simulink model "Coil_Gun_Simulations"  (R2020b)
settings: Solver=VariableStepAuto  StartTime=0.0  StopTime=1
model workspace (MAT data in the model file):
  Coil_Diameter = Simulink.Parameter
  Coil_Diameter.Value = 10
  Coil_Diameter.DataType = 'auto'
  Coil_Diameter.DocUnits = 'mm'
  Coil_Diameter.Dimensions = [1 1]
  Coil_Length = Simulink.Parameter
  Coil_Length.Value = 5
  Coil_Length.DataType = 'auto'
  Coil_Length.DocUnits = 'mm'
  Coil_Length.Dimensions = [1 1]
  Coil_Turns = Simulink.Parameter
  Coil_Turns.Value = 20
  Coil_Turns.DataType = 'auto'
  Coil_Turns.Dimensions = [1 1]
  Projectile_Density = Simulink.Parameter
  Projectile_Density.Value = 7850
  Projectile_Density.DataType = 'auto'
  Projectile_Density.DocUnits = 'kg/m^3'
  Projectile_Density.Dimensions = [1 1]
  Projectile_Diameter = Simulink.Parameter
  Projectile_Diameter.Value = 5
  Projectile_Diameter.DataType = 'auto'
  Projectile_Diameter.DocUnits = 'mm'
  Projectile_Diameter.Dimensions = [1 1]
  Projectile_Length = Simulink.Parameter
  Projectile_Length.Value = 5
  Projectile_Length.DataType = 'auto'
  Projectile_Length.DocUnits = 'mm'
  Projectile_Length.Dimensions = [1 1]
  u0 = Simulink.Parameter
  u0.Value = 1.256636e-06
  u0.DataType = 'auto'
  u0.DocUnits = 'N/A^2'
  u0.Dimensions = [1 1]
libraries: fl_lib x5, nesl_utility x4, ee_lib x3
settings Model: OrderedModelArguments=off  Creator=hanso  LastModifiedBy=hanso
settings SolverCC: ZeroCrossAlgorithm=Adaptive

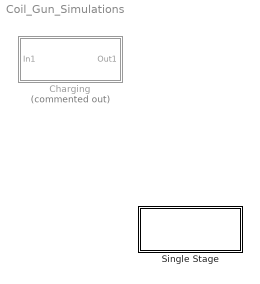
== system Coil_Gun_Simulations ==
  Charging : Subsystem  Commented=on
  Single Stage : Subsystem

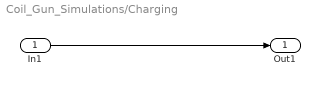
== system Coil_Gun_Simulations/Charging ==
  In1 : Inport
  Out1 : Outport
  wires:
  In1/1 -> Out1/1

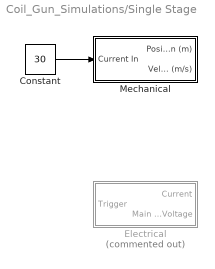
== system Coil_Gun_Simulations/Single Stage ==
  Constant : Constant  Value=30
  Electrical : Subsystem  Commented=on
  Mechanical : Subsystem
  wires:
  Constant/1 -> Mechanical/1(Current In)

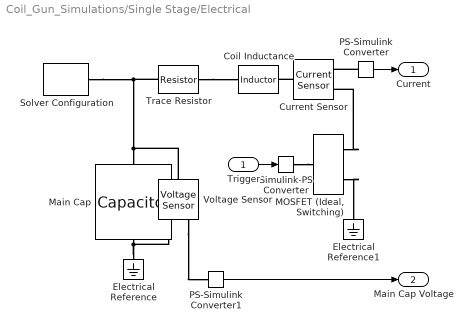
== system Coil_Gun_Simulations/Single Stage/Electrical ==
  Trigger : Inport
  Coil Inductance : ee_lib/Passive/Inductor  l=1e-03 H  L_tol=10  enable_L_tol=0  tol_distribution=1  nSigma=4  r=0 Ohm  g=1e-9 1/Ohm  enable_operating_limits=0  operating_limit_action=2  max_working_current=1 A  power_rating=1 W  enable_faults=0  fault_action=1  lambdaPercent=50  k_faulted=0.9999  turnsShort=0  openCct=0  groundShort=0  groundShortG=0 1/Ohm  tau_fault=1e-3 s  enable_temporal_fault=0  t_fault=1 s  enable_behavioral_fault=0  max_permissible_voltage=100 V  n_fail_on_voltage=1  max_permissible_current=1 A  t_fail_on_current=1 s  i_L_specify=off  i_L_priority=High  i_L=0 A  i_L_nominal_specify=off  i_L_nominal_unit=A  i_L_nominal_value=1
  Current Sensor : fl_lib/Electrical/Electrical Sensors/Current Sensor
  Electrical Reference : fl_lib/Electrical/Electrical Elements/Electrical Reference
  Electrical Reference1 : fl_lib/Electrical/Electrical Elements/Electrical Reference
  "MOSFET (Ideal, Switching)" : ee_lib/Semiconductors & Converters/MOSFET (Ideal, Switching)  Rds=0.01 Ohm  Goff=1e-6 1/Ohm  Vth=2 V  diode_param=ee.enum.converters.protectiondiode.none  diode_Vf=0.8 V  diode_Ron=0.001 Ohm  diode_Goff=1e-5 1/Ohm  diode_C=50e-9 F  diode_iRM=-235 A  diode_iF=300 A  diode_idot=-50 A/us  diode_trr_param=ee.enum.converters.diodetrr.trr_factor  diode_trr_factor=3  diode_trr=15 us  diode_Qrr=1500 s*uA  thermal_loss_option=ee.enum.converters.thermalLossOption.constantvalues  Von_data=[0, 1.1, 1.3, 1.45, 1.75, 2.25, 2.7; 0, 1, 1.15, 1.35, 1.7, 2.35, 3] V  Eon_data=[0, .29, 1.43, 2.86, 5.71, 13.14, 22.86; 0, .57, 2.63, 5.14, 10.29, 20.57, 30.29] * 1e-3 J  Eoff_data=[0, .21, 1.07, 2.14, 4.29, 9.86, 17.14; 0, .43, 1.97, 3.86, 7.71, 15.43, 22.71] * 1e-3 J  Tj=[298.15, 398.15] K  Iout_data=[0, 10, 50, 100, 200, 400, 600] A  Eon_scalar=22.86e-3 J  Eoff_scalar=17.14e-3 J  Voff=300 V  Iout_scalar=600 A  diodeModelType=ee.enum.converters.diodeModelType.pwl  diode_IfMat=[.07, .12, .19, 1.75, 4.24, 7.32, 11.2; .16, .3, .72, 2.14, 4.02, 6.35, 9.12] A  diode_TjVec=[25, 125] degC  diode_VfVec=[.5, .7, .9, 1.3, 1.7, 2.1, 2.5] V  thermal_network_parameterization=ee.enum.thermalNetworkTopology.external  Rth=[.03, .2] K/W  Rth_Foster=[.03, .2] K/W  thermal_mass_parameterization=ee.enum.thermalNetwork.timeconstant  thermal_mass=[3, 25] J/K  thermal_mass_Foster=[33, 50] J/K  thermal_time_constant=[.1, 5] s  thermal_time_constant_Foster=[1, 10] s  thermal_mass_initial_temperatures=[25, 25] degC  junction_thermal_mass=0.1 J/K  Tau=1e-4 s  vT_specify=off  vT_priority=None  vT=0 V  vT_nominal_specify=off  vT_nominal_unit=V  vT_nominal_value=1  Qj_specify=off  Qj_priority=None  Qj=0 W  Qj_nominal_specify=off  Qj_nominal_unit=W  Qj_nominal_value=1  junction_temperature_specify=off  junction_temperature_priority=None  junction_temperature=25 degC  junction_temperature_nominal_specify=off  junction_temperature_nominal_unit=degC  junction_temperature_nominal_value=1
  Main Cap : ee_lib/Passive/Capacitor  cap_option=0  c=2400e-6 F  Cvec=[1e-05, 1e-06] F  Vvec=[0, 10] V  CV_table_symmetry=1  f_vec=[1, 10] kHz  DFext_vec=[.8, 1.2]  C_tol=5  enable_C_tol=0  tol_distribution=1  nSigma=4  r=1e-6 Ohm  g=0 1/Ohm  averaging_period=0 s  enable_operating_limits=0  operating_limit_action=2  max_working_voltage_range=[-25, 25] V  power_rating=1 W  enable_faults=0  fault_action=1  Cscale_faulted=100  R_faulted=1e-3 Ohm  G_faulted=0 1/Ohm  tau_fault=1e-3 s  enable_temporal_fault=0  t_fault=1 s  enable_behavioral_fault=0  max_permissible_voltage_range=[-100, 100] V  t_fail_on_voltage=1 s  i_specify=off  i_priority=None  i=0 A  i_nominal_specify=off  i_nominal_unit=A  i_nominal_value=1  v_specify=off  v_priority=None  v=10 V  v_nominal_specify=off  v_nominal_unit=V  v_nominal_value=1  vc_specify=on  vc_priority=High  vc=10 V  vc_nominal_specify=off  vc_nominal_unit=V  vc_nominal_value=1
  PS-Simulink Converter : nesl_utility/PS-Simulink Converter  PhysicalDomain=network_engine_domain  SubClassName=ps_output  LeftPortType=input  RightPortType=output  PseudoPeriodic=off  Frequencies=[]  Unit=inherit  AffineConversion=off
  PS-Simulink Converter1 : nesl_utility/PS-Simulink Converter  PhysicalDomain=network_engine_domain  SubClassName=ps_output  LeftPortType=input  RightPortType=output  PseudoPeriodic=off  Frequencies=[]  Unit=inherit  AffineConversion=off
  Simulink-PS Converter : nesl_utility/Simulink-PS Converter  PhysicalDomain=network_engine_domain  SubClassName=ps_input  LeftPortType=input  RightPortType=output  PseudoPeriodic=off  Frequencies=[]  NoiseDistribution=none  NoiseParameters=[]  Unit=1  AffineConversion=off  FilteringAndDerivatives=provide  SimscapeFilterOrder=1  InputFilterTimeConstant=0.001  UdotUserProvided=0
  Solver Configuration : nesl_utility/Solver Configuration  PhysicalDomain=network_engine_domain  SubClassName=solver  LeftPortType=input  RightPortType=generic  Tones=[]  Harmonics=[]  SimulateNoise=off  Profile=off  UseLocalSampling=off  EnableSwitchedLinearOptims=on  FrequencyDomain=off  UseCCode=off  RelTol=0.001  AbsTol=1e-06  MinStep=1e-09  ToWorkspace=off  RevertToSquareIcSolve=off  NumHomotopyIterations=100  PhasorMode=off  PhasorModeNumHarmonics=1  DoDC=off  ResidualTolerance=1e-09  UseLocalSolver=off  LocalSolverChoice=NE_TRAPEZOIDAL_ADVANCER  LocalSolverSampleTime=1e-6  DoFixedCost=off  MaxNonlinIter=3  MaxModeIter=2  ComputeImpulses=off  ImpulseIterations=2  LinearAlgebra=auto  EquationFormulation=NE_TIME_EF  DelaysMemoryBudget=1024  AutomaticFiltering=off  FilteringTimeConstant=0.001  PartitionStorageMethod=AS_NEEDED  PartitionMemoryBudget=1024  PartitionMethod=ROBUST
  Trace Resistor : fl_lib/Electrical/Electrical Elements/Resistor  R=1 Ohm  i_specify=off  i_priority=None  i=0 A  i_nominal_specify=off  i_nominal_unit=A  i_nominal_value=1  v_specify=off  v_priority=None  v=0 V  v_nominal_specify=off  v_nominal_unit=V  v_nominal_value=1
  Voltage Sensor : fl_lib/Electrical/Electrical Sensors/Voltage Sensor
  Current : Outport
  Main Cap Voltage : Outport  Port=2
  wires:
  PS-Simulink Converter/1 -> Current/1
  PS-Simulink Converter1/1 -> Main Cap Voltage/1
  Trigger/1 -> Simulink-PS Converter/1
  connections:
  Solver Configuration/RConn1 -- Trace Resistor/LConn1 -- Voltage Sensor/LConn1 -- Main Cap/LConn1
  Main Cap/RConn1 -- Voltage Sensor/RConn2 -- Electrical Reference/LConn1
  "MOSFET (Ideal, Switching)"/RConn2 -- Electrical Reference1/LConn1
  Current Sensor/LConn1 -- Coil Inductance/RConn1
  "MOSFET (Ideal, Switching)"/RConn1 -- Current Sensor/RConn2
  PS-Simulink Converter/LConn1 -- Current Sensor/RConn1
  Voltage Sensor/RConn1 -- PS-Simulink Converter1/LConn1
  Simulink-PS Converter/RConn1 -- "MOSFET (Ideal, Switching)"/LConn1
  Trace Resistor/RConn1 -- Coil Inductance/LConn1

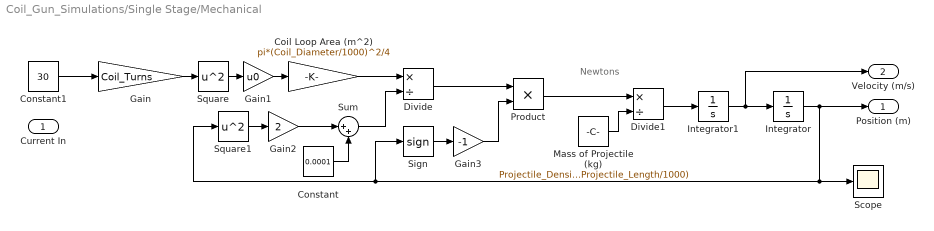
== system Coil_Gun_Simulations/Single Stage/Mechanical ==
  note: Newtons
  Current In : Inport
  Coil Loop Area (m^2) : Gain  Gain=pi*(Coil_Diameter/1000)^2/4
  Constant : Constant  Value=0.0001
  Constant1 : Constant  Value=30
  Divide : Product  Inputs=*/
  Divide1 : Product  Inputs=*/
  Gain : Gain  Gain=Coil_Turns
  Gain1 : Gain  Gain=u0
  Gain2 : Gain  Gain=2
  Gain3 : Gain  Gain=-1
  Integrator : Integrator  InitialCondition=-0.002
  Integrator1 : Integrator
  Mass of Projectile (kg) : Constant  Value=Projectile_Density*pi*(Projectile_Diameter/1000)^2/4*(Projectile_Length/1000)
  Product : Product
  Scope : Scope
  Sign : Signum
  Square : Math  Operator=square  SaturateOnIntegerOverflow=on
  Square1 : Math  Operator=square  SaturateOnIntegerOverflow=on
  Sum : Sum  Inputs=|++
  Position (m) : Outport
  Velocity (m/s) : Outport  Port=2
  wires:
  Gain/1 -> Square/1
  Square/1 -> Gain1/1
  Gain1/1 -> Coil Loop Area (m^2)/1
  Coil Loop Area (m^2)/1 -> Divide/1
  Square1/1 -> Gain2/1
  Integrator/1 -> Position (m)/1, Scope/1, Sign/1, Square1/1
  Integrator1/1 -> Velocity (m/s)/1, Integrator/1
  Product/1 -> Divide1/1
  Mass of Projectile (kg)/1 -> Divide1/2
  Divide1/1 -> Integrator1/1
  Divide/1 -> Product/1
  Constant1/1 -> Gain/1
  Gain2/1 -> Sum/1
  Constant/1 -> Sum/2
  Sum/1 -> Divide/2
  Sign/1 -> Gain3/1
  Gain3/1 -> Product/2
